simulink model "Reaching_mouse"  (R2024b)
settings: Solver=FixedStepDiscrete  StartTime=0.0  StopTime=inf  FixedStep=0.001  RelTol=1e-3
undefined symbols (not defined in the file): get
libraries: PhanTorque_3Dof_Library_64Bits x1, vrlib x1
settings Model: Creator=carlos.aldana  LastModifiedBy=danie
settings SolverCC: AlgebraicLoopSolver=TrustRegion
settings DataIOCC: LimitDataPoints=on  SaveFormat=Array  ReturnWorkspaceOutputs=off
settings OptimizationCC: BlockReduction=off  BooleanDataType=off  LifeSpan=inf
settings DebuggingCC: SaveWithParameterizedLinksMsg=none  UnderspecifiedInitializationDetection=Classic  MergeDetectMultiDrivingBlocksExec=none  SignalResolutionControl=TryResolveAllWithWarning  UnconnectedInputMsg=warning  UnconnectedOutputMsg=warning  UnconnectedLineMsg=warning  AllowSymbolicDim=off  SFUnexpectedBacktrackingDiag=warning  SFNoUnconditionalDefaultTransitionDiag=warning  SFExecutionAtInitializationDiag=none  ArithmeticOperatorsInVariantConditions=warning
settings HardwareCC: ProdBitPerPointer=32  ProdBitPerSizeT=32  ProdBitPerPtrDiffT=32  ProdLargestAtomicFloat=None  ProdIntDivRoundTo=Undefined  ProdEndianess=Unspecified  ProdWordSize=32  ProdHWDeviceType=32-bit Generic  TargetUnknown=on
settings ModelReferenceCC: EnableRefExpFcnMdlSchedulingChecks=on  PropagateSignalLabelsOutOfModel=off
settings SFSimCC: SimUseLocalCustomCode=off  CustomCodeUndefinedFunction=UseInterfaceOnly
settings RTWCC: RTWUseLocalCustomCode=off  GPUComputeCapability=3.5  DLArmComputeVersion=19.05
settings CodeAppCC: StateflowObjectComments=on
settings GRTTargetCC: TargetLangStandard=C89/C90 (ANSI)
settings ConfigComp: CovMetricSettings=dw  CovSaveCumulativeToWorkspaceVar=on  CovSaveSingleToWorkspaceVar=on  CovExternalEMLEnable=off  CovSFcnEnable=off

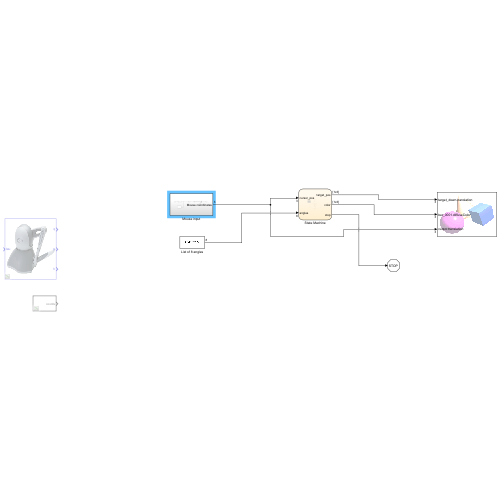
[thumbnail: Simulink's stored preview of the top-level diagram]
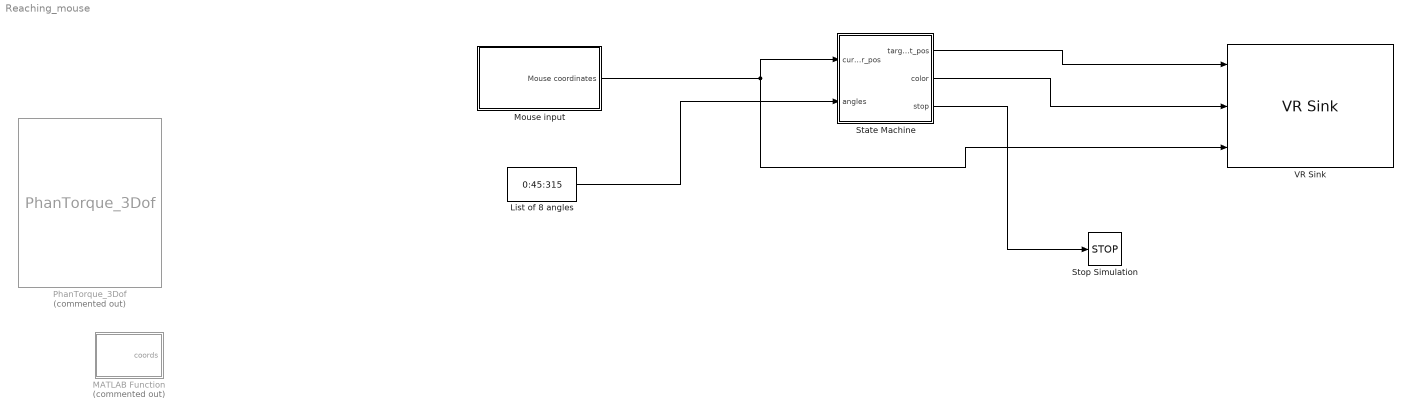
== system Reaching_mouse ==
  List of 8 angles : Constant  Value=0:45:315
  MATLAB Function : MATLAB Function  Commented=on  TreatAsAtomicUnit=on
  Mouse input : Subsystem
  PhanTorque_3Dof : PhanTorque_3Dof_Library_64Bits/PhanTorque_3Dof  Commented=on  Haptic_Name='Default Device'
  State Machine : Stateflow chart  TreatAsAtomicUnit=on
  Stop Simulation : Stop
  VR Sink : vrlib/VR Sink  InstantiateOnLoad=on  SampleTime=0.1  ViewEnable=on  RemoteChange=off  RemoteView=off  FieldsWritten=target_down.translation.3.1.1.double#ber_0001.diffuseColor.3.1.1.double#cursor.translation.3.1.1.double  WorldFileName=VR_centerAndTarget.wrl  AutoView=off  VideoDimensions=[]  AllowVariableSize=off
  wires:
  Mouse input/1(Mouse coordinates) -> State Machine/1(cursor_pos), VR Sink/3
  List of 8 angles/1 -> State Machine/2(angles)
  State Machine/1(target_pos) -> VR Sink/1
  State Machine/2(color) -> VR Sink/2
  State Machine/3(stop) -> Stop Simulation/1

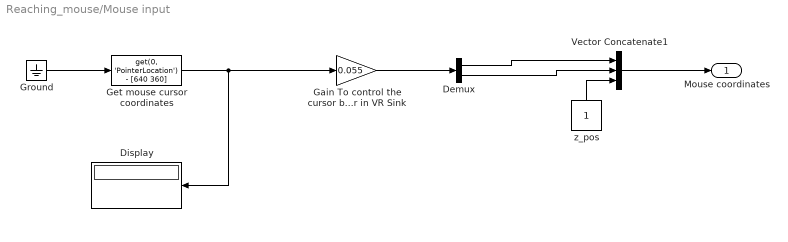
== system Reaching_mouse/Mouse input ==
  Demux : Demux  Outputs=2
  Display : Display
  Gain To control the cursor better in VR Sink : Gain  Gain=0.055
  Get mouse cursor coordinates : MATLABFcn  MATLABFcn=get(0, 'PointerLocation') - [640 360]  OutputDimensions=2
  Ground : Ground
  Vector Concatenate1 : Concatenate  NumInputs=3
  z_pos : Constant
  Mouse coordinates : Outport
  wires:
  Gain To control the cursor better in VR Sink/1 -> Demux/1
  Demux/2 -> Vector Concatenate1/2
  Ground/1 -> Get mouse cursor coordinates/1
  Get mouse cursor coordinates/1 -> Display/1, Gain To control the cursor better in VR Sink/1
  Demux/1 -> Vector Concatenate1/1
  Vector Concatenate1/1 -> Mouse coordinates/1
  z_pos/1 -> Vector Concatenate1/3

== stateflow chart Reaching_mouse/State Machine ==
  state Initializing
    entry:
    ext_loop = 1;
    radius = 10;
    counter_point = 1;
    %target_pos = [0 0 0];
  state RandomAngleList
    entry:
    random_angle_list = randomAngle(angles);
  state SpawnTarget
    entry:
    color = [1 0 0];
    target_pos = computeTargetPose(random_angle_list(counter_point), radius);
  state ReachingTarget
    entry:
    color = [0 1 0];
  state SpawnHome
    entry:
    target_pos = [0 0 0]; %Home pos
    color = [0.5 0 1];
  state ReachingHome
    entry:
    color = [0.9 0.5 0.95];
  state Finish
    stop = 1;
  (default) -> Initializing [order 2]
  (default) -> Initializing [order 1]
  Initializing -> RandomAngleList
  ReachingHome -> RandomAngleList [order 3] : after(2, sec)[counter_point == 8 & sqrt((target_pos(1)-cursor_pos(1))^2 + (target_pos(2)-cursor_pos(2))^2) < 0.4]{ext_loop = ext_loop+1}
  RandomAngleList -> SpawnTarget
  ReachingHome -> SpawnTarget [order 4] : after(2, sec)[counter_point ~= 8 & sqrt((target_pos(1)-cursor_pos(1))^2 + (target_pos(2)-cursor_pos(2))^2) <= 0.4]{counter_point = counter_point + 1}
  SpawnTarget -> ReachingTarget : [sqrt((target_pos(1)-cursor_pos(1))^2 + (target_pos(2)-cursor_pos(2))^2) <= 0.4]
  ReachingTarget -> SpawnTarget [order 1] : [sqrt((target_pos(1)-cursor_pos(1))^2 + (target_pos(2)-cursor_pos(2))^2) > 0.4]
  ReachingTarget -> SpawnHome [order 2] : after(1, sec)[sqrt((target_pos(1)-cursor_pos(1))^2 + (target_pos(2)-cursor_pos(2))^2) <= 0.4]
  SpawnHome -> ReachingHome : [sqrt((target_pos(1)-cursor_pos(1))^2 + (target_pos(2)-cursor_pos(2))^2) <= 0.4]
  ReachingHome -> SpawnHome [order 1] : [sqrt((target_pos(1)-cursor_pos(1))^2 + (target_pos(2)-cursor_pos(2))^2) > 0.4]
  ReachingHome -> Finish [order 2] : [ext_loop == 10 & counter_point == 8]
  data: angle_list function_input; random_angle_list function_output; single_angle function_input; point_coordinates function_output; radius function_input; cursor_pos input; target_pos output; counter local; time local; target_color local; radius local; angle local; angles input; color output; stop output; ext_loop local; counter_point local; random_angle_list local
  function random_angle_list = randomAngle(angle_list):
    | function random_angle_list = randomAngle(angle_list)
    |     % size_list = length(angle_list);
    |     
    |     % % To compute a new seed at each call
    |     % rng('shuffle');
    |     % % Compute a new permutation at each call using the seed
    |     % random_index = randperm(size_list);
    |     % 
    |     % % Initialize the new list with the lenght of al
    |     % new_list = zeros(size_list, 1);
    |     % 
    |     % for i = 1:size_list
    |     %     % Assign the element of al in random order
    |     %     new_list(i) = angle_list(random_index(i));
    |     % end
    |     % 
    |     % random_list = new_list;
    | 
    |     % To compute a new seed at each call
    |     rng('shuffle');
    |     random_indeces = randperm(length(angle_list));
    |     random_angle_list = angle_list(random_indeces);
    | 
    | 
    | end
  function point_coordinates = computeTargetPose(single_angle, radius):
    | function point_coordinates = computeTargetPose(single_angle, radius)
    |     theta = deg2rad(single_angle);
    |     % Compute the coordinates of the points in the circumference
    |     x = radius * cos(theta);
    |     y = radius * sin(theta);
    |     z = 0; % lower than mouse cursor
    | 
    |     point_coordinates = [x y z];
    | end

== matlab function Reaching_mouse/MATLAB Function ==
  data: coords output
function coords = get_pointer_coordinates
    coords = get(0, 'PointerLocation');
